simulink model "mechanical_model_sw_input"  (R2019b)
settings: Solver=FixedStepAuto  StartTime=0.0  StopTime=10  FixedStep=1e-3  RelTol=1e-3
undefined symbols (not defined in the file or in its folder): tf2_1, tf2_2
settings Model: Creator=Guido  LastModifiedBy=pietr

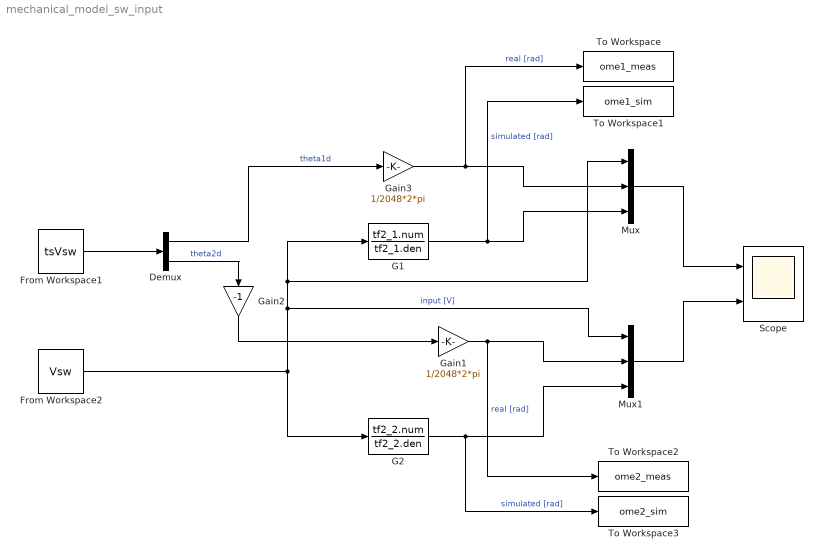
== system mechanical_model_sw_input ==
  Demux : Demux  Outputs=2
  From Workspace1 : FromWorkspace  VariableName=tsVsw  SampleTime=0
  From Workspace2 : FromWorkspace  VariableName=Vsw  SampleTime=0
  G1 : TransferFcn  Numerator=tf2_1.num  Denominator=tf2_1.den
  G2 : TransferFcn  Numerator=tf2_2.num  Denominator=tf2_2.den
  Gain1 : Gain  Gain=1/2048*2*pi
  Gain2 : Gain  Gain=-1
  Gain3 : Gain  Gain=1/2048*2*pi
  Mux : Mux  Inputs=3
  Mux1 : Mux  Inputs=3
  Scope : Scope  NumInputPorts=2
  To Workspace : ToWorkspace  VariableName=ome1_meas  SampleTime=-1
      settings: Save2DSignal=2-D array (concatenate along first dimension)
  To Workspace1 : ToWorkspace  VariableName=ome1_sim  SampleTime=-1
      settings: Save2DSignal=2-D array (concatenate along first dimension)
  To Workspace2 : ToWorkspace  VariableName=ome2_meas  SampleTime=-1
      settings: Save2DSignal=2-D array (concatenate along first dimension)
  To Workspace3 : ToWorkspace  VariableName=ome2_sim  SampleTime=-1
      settings: Save2DSignal=2-D array (concatenate along first dimension)
  wires:
  Demux/1 -> Gain3/1  "theta1d"
  Demux/2 -> Gain2/1  "theta2d"
  Mux/1 -> Scope/1
  Mux1/1 -> Scope/2
  Gain2/1 -> Gain1/1
  G1/1 -> To Workspace1/1, Mux/3  "simulated [rad]"
  From Workspace1/1 -> Demux/1
  Gain3/1 -> To Workspace/1, Mux/2  "real [rad]"
  From Workspace2/1 -> Mux/1, G1/1, Mux1/1, G2/1  "input [V]"
  G2/1 -> To Workspace3/1, Mux1/3  "simulated [rad]"
  Gain1/1 -> To Workspace2/1, Mux1/2  "real [rad]"
